simulink model "tqdtqr_rebuild_V3"  (R2021b)
settings: Solver=VariableStepAuto  StartTime=0.0  StopTime=10.0  RelTol=1e-3
undefined symbols (not defined in the file): ATQD_AfterTqMinGain_X_Deg, ATQD_APSCreepBaseTqD_X_kph, ATQD_APSCreepBaseTqD_Y_Deg, ATQD_APSCreepBaseTqR_X_kph, ATQD_APSCreepBaseTqR_Y_Deg, ATQD_APSCreepIterm_X_kph, ATQD_APSCreepIterm_Y_kph, ATQD_APSCreepPterm_X_kph, ATQD_APSCreepPterm_Y_kph, ATQD_APSDecReq_X_kph, ATQD_APSDecReq_Y_mps2, ATQD_APSDecReqCMD_X_kph, ATQD_APSDecReqTs_X_pct, ATQD_APSDecTimeGain_X_Deg, ATQD_APSDecTimeGain_Y_s, ATQD_APSReqLowSpd_X_Deg, ATQD_AutoHoldReleaseBPS_X_Deg, ATQD_AWDLoadTrqnsGain_X_kg, ATQD_AWDLoadTrqnsGain_Y_pct, ATQD_BOSEnBPSPosn_X_kph, ATQD_BOSMap_X_rpm, ATQD_BOSMap_Y_pct, ATQD_CreepBaseTqD_X_kph, ATQD_CreepBaseTqD_Y_Deg, ATQD_CreepBaseTqR_X_kph, ATQD_CreepBaseTqR_Y_Deg, ATQD_CreepBPSDisPosn_X_Deg, ATQD_CreepBPSDisPosnR_X_Deg, ATQD_CreepBPSEnPosn_X_Deg, ATQD_CreepBPSEnPosnR_X_Deg, ATQD_CreepDeltaTq_X_kph, ATQD_CreepIterm_X_kph, ATQD_CreepIterm_Y_kph, ATQD_CreepItermMaxLimit_X_pct, ATQD_CreepPreloadTime_X_kph, ATQD_CreepPreloadTq_X_kph, ATQD_CreepPreloadTq_Y_s, ATQD_CreepProtTq_X_Deg, ATQD_CreepPterm_X_kph, ATQD_CreepPterm_Y_kph, ATQD_CreepRrTqSpRat_X_rpm, ATQD_CreepRrTqSpRat_Y_Nm, ATQD_CreepTargetSpdD_X_pct, ATQD_CreepTargetSpdR_X_pct, ATQD_CreepUpLimitTq_X_rpm, ATQD_DecIneOPDHoldEnDelay_X_Deg, ATQD_DecIneOPDHoldEnDelay_Y_bar, ATQD_ECOTqMapD_X_rpm, ATQD_ECOTqMapD_Y_pct, ATQD_EMTqMapD_X_rpm, ATQD_EMTqMapD_Y_pct, ATQD_EOPDTqMapDCon_X_rpm, ATQD_EOPDTqMapDCon_Y_Deg, ATQD_EstInitVehWeight_X_c, ATQD_FAfterTqCMDGain_X_rpm, ATQD_FAfterTqCMDGain_Y_pct, ATQD_ForceLowSpd_X_Deg, ATQD_ForcePLimitSpd_X_Deg, ATQD_FrLossMAPLowV_X_rpm, ATQD_FrLossMAPLowV_Y_Nm ... (+949)
libraries: simulink x235, hcu_lib x208, tqr x63, tqd x6
(part 3 of 37)

== system tqdtqr_rebuild_V3/SCP_Out ==
  BInpConvert_outputs : Inport
  BMain_outputs : Inport  Port=2
  BOutpConvert_outputs : Inport  Port=3
  Bus Selector : BusSelector  OutputSignals=VTQD_GearActualPosn_enum,VTQD_ParkRequest_flg,VTQD_PBWLockTO_flg,VTQD_PBWUnlockTO_flg,VTQD_TqSourceFr_enum,VTQD_TqSourceRr_enum,VTQD_TqTargetShaftSpd_rpm,VTQD_LimpHomeAct_flg,VTQD_RollRegenEnable_flg,VTQD_EVDriveMode_enum,VTQD_EVDriveModeValid_flg,VTQD_ShiftGearPosn_enum,VTQD_FrActvDmpDisabReq_flg,VTQD_RrActvDmpDisabReq_flg,VTQD_CreepEnable_flg,VTQD_LoSpdBrkCtrl_flg,VTQD_LowIdleAccPedal_flg,VTQD_APSStaSys_enum,VTQD_APSReq_enum,VTQD_APSDecReqA_flg,VTQD_APSDecReq_mps2,VTQD_EstVehWeightResult_kg,VTQD_BOSEnable_flg,VTQD_CreepON_flg,VTQD_PreLoadHold_flg,VTQD_PreLoadPreEn_flg,VTQD_CreepPrLoadEnable_flg,VTQD_RDCActive_enum,VTQD_DriveProtEn_flg,VTQD_ActParkRequest_flg,VTQD_RegenTqLimitEn_flg,VTQD_PedAccTqEn_flg,VTQD_IVIPwrLockSta_enum,VTQD_WhlTqCapGenFr_Nm,VTQD_WhlTqCapGenRr_Nm,VTQD_OPDHoldLamp_flg,VTQD_RegenMode_enum,VTQD_SaveRegenMode_enum,VTQD_FDCVCURegenMode_enum,VTQD_SpdCtrlMode_enum,VTQD_SpdCtrlSta_flg,VTQD_SetSpd_kph,VTQD_SWCCancelSta_flg,VTQD_SWCSetdownSta_flg,VTQD_SWCResUpSta_flg,VTQD_CreepBaseTqD_Nm,VTQD_VehActSpd_kph,VTQD_BrkSwSta_flg,VTQD_SWC2CancelSta_flg,VTQD_SWC2SetdownSta_flg,VTQD_SWC2ResUpSta_flg,VTQD_SWC2LADASSta_flg,VTQD_SpdLim4SetSpd_raw32,VTQD_MaxWhlSlideRate_pct,VTQD_MinWhlSlideRate_pct,VTQD_LeftSlideRate_pct,VTQD_RightSlideRate_pct,VTQD_FrontSlideRate_pct,VTQD_RearSlideRate_pct,VTQD_TrailerDisOPDSta_flg,VTQD_ComboKeyPreEn_flg,VTQD_ComboKeyEn_flg,VTQD_SysMode_enum,VTQD_WhlTqCapMotFr_Nm,VTQD_WhlTqCapMotRr_Nm,VTQD_FrShaftSpd_rpm,VTQD_RrShaftSpd_rpm,VTQD_EPBCarWashMode_flg,VTQD_IVIRockModeEn_flg,VTQD_ForceP_flg,VTQD_SlideRegenLimTq_Nm,VTQD_SimSoundCmd_pct,VTQD_SimSouWaveReq_pct,VTQD_RockModeTCSReq_flg,VTQD_TMEnOutpTqSta_enum,VTQR_RShaftSpdTqLimLow_flg,VTQR_RTimerTqLimLow_flg,VTQR_FShaftSpdTqLimLow_flg,VTQR_FTimerTqLimLow_flg,VTQR_FrFirstOrderInpTs_c,VTQR_RrFirstOrderInpTs_c,VTQR_FrRateLimitInc_Nm,VTQR_FrRateLimitDec_Nm,VTQR_RrRateLimitInc_Nm,VTQR_RrRateLimitDec_Nm,VTQR_FrTqZeroTransLowBound_Nm,VTQR_RrTqZeroTransUpBound_Nm,VTQR_FrTqZeroTrans_enum,VTQR_RrTqZeroTrans_enum
  Bus Selector1 : BusSelector  OutputSignals=VTQD_DriverWhlTqDem_Nm,VTQD_AfterAvailableTqDemFr_Nm,VTQD_AfterAvailableTqDemRr_Nm,VTQD_CoordWhlTqDemFr_Nm,VTQD_CoordWhlTqDemRr_Nm,VTQR_FrTMTqReq_Nm,VTQR_RrTMTqReq_Nm,VTQR_ActualFEDUWhlTqReq_Nm,VTQR_ActualREDUWhlTqReq_Nm,VTQR_NoABSFEDUWhlTqReq_Nm,VTQR_NoABSREDUWhlTqReq_Nm
  Bus Selector2 : BusSelector  OutputSignals=VTQD_FrEDUAvailBrkRgnTq_Nm,VTQD_RrEDUAvailBrkRgnTq_Nm,VTQD_PButtonSta_enum,VTQD_FrRgnDecrSta_flg,VTQD_RrRgnDecrSta_flg,VTQD_DriverWhlTqDemFr_Nm,VTQD_DriverWhlTqDemRr_Nm,VTQD_FrEDUActTq_Nm,VTQD_RrEDUActTq_Nm,VTQD_FrEDURolRgnTq_Nm,VTQD_RrEDURolRgnTq_Nm,VTQD_FrEDUSpd_rpm,VTQD_RrEDUSpd_rpm,VTQD_FrEDUSpdValid_flg,VTQD_FrEDUAvailBrkRgnTqV_flg,VTQD_RrEDUSpdValid_flg,VTQD_RrEDUAvailBrkRgnTqV_flg,VTQD_RgnAbnorSta_flg,VTQD_PTCSPermSta_flg,VTQD_FrRgnPermSta_flg,VTQD_RrRgnPermSta_flg,VTQD_ExternalTqAllow_flg,VTQD_FrIdcMin_A,VTQD_FrIdcMax_A,VTQD_FrUdcMin_V,VTQD_FrUdcMax_V,VTQD_RrIdcMin_A,VTQD_RrIdcMax_A,VTQD_RrUdcMin_V,VTQD_RrUdcMax_V,VTQD_CrashDetd_flg,VTQD_DiagHCrash_flg,VTQD_ReBrakeLPReq_flg,VTQD_ExtShftAllow_flg,VTQD_EquivAccPedalSWSta_flg,VTQD_ExtDoorAllow_flg,VTQD_RegenLimIndSta_flg,VTQD_SetSpdLimWarn_flg,VTQD_CrashUnlockReq_flg,VTQD_CTDCtrl_enum
  Bus Creator : BusCreator  Inputs=140
  BDrivingControl_outputs : Outport
  wires:
  BInpConvert_outputs/1 -> Bus Selector/1
  BMain_outputs/1 -> Bus Selector1/1
  BOutpConvert_outputs/1 -> Bus Selector2/1
  Bus Selector/1 -> Bus Creator/1  "<VTQD_GearActualPosn_enum>"
  Bus Selector/2 -> Bus Creator/2  "<VTQD_ParkRequest_flg>"
  Bus Selector/3 -> Bus Creator/3  "<VTQD_PBWLockTO_flg>"
  Bus Selector/4 -> Bus Creator/4  "<VTQD_PBWUnlockTO_flg>"
  Bus Selector/5 -> Bus Creator/5  "<VTQD_TqSourceFr_enum>"
  Bus Selector/6 -> Bus Creator/6  "<VTQD_TqSourceRr_enum>"
  Bus Selector/7 -> Bus Creator/7  "<VTQD_TqTargetShaftSpd_rpm>"
  Bus Selector/8 -> Bus Creator/8  "<VTQD_LimpHomeAct_flg>"
  Bus Selector/9 -> Bus Creator/9  "<VTQD_RollRegenEnable_flg>"
  Bus Selector/10 -> Bus Creator/10  "<VTQD_EVDriveMode_enum>"
  Bus Selector/11 -> Bus Creator/11  "<VTQD_EVDriveModeValid_flg>"
  Bus Selector/12 -> Bus Creator/12  "<VTQD_ShiftGearPosn_enum>"
  Bus Selector/13 -> Bus Creator/13  "<VTQD_FrActvDmpDisabReq_flg>"
  Bus Selector/14 -> Bus Creator/14  "<VTQD_RrActvDmpDisabReq_flg>"
  Bus Selector/15 -> Bus Creator/15  "<VTQD_CreepEnable_flg>"
  Bus Selector/16 -> Bus Creator/16  "<VTQD_LoSpdBrkCtrl_flg>"
  Bus Selector/17 -> Bus Creator/17  "<VTQD_LowIdleAccPedal_flg>"
  Bus Selector/18 -> Bus Creator/18  "<VTQD_APSStaSys_enum>"
  Bus Selector/19 -> Bus Creator/19  "<VTQD_APSReq_enum>"
  Bus Selector/20 -> Bus Creator/20  "<VTQD_APSDecReqA_flg>"
  Bus Selector/21 -> Bus Creator/21  "<VTQD_APSDecReq_mps2>"
  Bus Selector/22 -> Bus Creator/22  "<VTQD_EstVehWeightResult_kg>"
  Bus Selector/23 -> Bus Creator/23  "<VTQD_BOSEnable_flg>"
  Bus Selector/24 -> Bus Creator/24  "<VTQD_CreepON_flg>"
  Bus Selector/25 -> Bus Creator/25  "<VTQD_PreLoadHold_flg>"
  Bus Selector/26 -> Bus Creator/26  "<VTQD_PreLoadPreEn_flg>"
  Bus Selector/27 -> Bus Creator/27  "<VTQD_CreepPrLoadEnable_flg>"
  Bus Selector/28 -> Bus Creator/28  "<VTQD_RDCActive_enum>"
  Bus Selector/29 -> Bus Creator/29  "<VTQD_DriveProtEn_flg>"
  Bus Selector/30 -> Bus Creator/30  "<VTQD_ActParkRequest_flg>"
  Bus Selector/31 -> Bus Creator/31  "<VTQD_RegenTqLimitEn_flg>"
  Bus Selector/32 -> Bus Creator/32  "<VTQD_PedAccTqEn_flg>"
  Bus Selector/33 -> Bus Creator/33  "<VTQD_IVIPwrLockSta_enum>"
  Bus Selector/34 -> Bus Creator/34  "<VTQD_WhlTqCapGenFr_Nm>"
  Bus Selector/35 -> Bus Creator/35  "<VTQD_WhlTqCapGenRr_Nm>"
  Bus Selector/36 -> Bus Creator/36  "<VTQD_OPDHoldLamp_flg>"
  Bus Selector/37 -> Bus Creator/37  "<VTQD_RegenMode_enum>"
  Bus Selector/38 -> Bus Creator/38  "<VTQD_SaveRegenMode_enum>"
  Bus Selector/39 -> Bus Creator/39  "<VTQD_FDCVCURegenMode_enum>"
  Bus Selector/40 -> Bus Creator/40  "<VTQD_SpdCtrlMode_enum>"
  Bus Selector/41 -> Bus Creator/41  "<VTQD_SpdCtrlSta_flg>"
  Bus Selector/42 -> Bus Creator/42  "<VTQD_SetSpd_kph>"
  Bus Selector/43 -> Bus Creator/43  "<VTQD_SWCCancelSta_flg>"
  Bus Selector/44 -> Bus Creator/44  "<VTQD_SWCSetdownSta_flg>"
  Bus Selector/45 -> Bus Creator/45  "<VTQD_SWCResUpSta_flg>"
  Bus Selector/46 -> Bus Creator/46  "<VTQD_CreepBaseTqD_Nm>"
  Bus Selector/47 -> Bus Creator/47  "<VTQD_VehActSpd_kph>"
  Bus Selector/48 -> Bus Creator/48  "<VTQD_BrkSwSta_flg>"
  Bus Selector/49 -> Bus Creator/49  "<VTQD_SWC2CancelSta_flg>"
  Bus Selector/50 -> Bus Creator/50  "<VTQD_SWC2SetdownSta_flg>"
  Bus Selector/51 -> Bus Creator/51  "<VTQD_SWC2ResUpSta_flg>"
  Bus Selector/52 -> Bus Creator/52  "<VTQD_SWC2LADASSta_flg>"
  Bus Selector/53 -> Bus Creator/53  "<VTQD_SpdLim4SetSpd_raw32>"
  Bus Selector/54 -> Bus Creator/54  "<VTQD_MaxWhlSlideRate_pct>"
  Bus Selector/55 -> Bus Creator/55  "<VTQD_MinWhlSlideRate_pct>"
  Bus Selector/56 -> Bus Creator/56  "<VTQD_LeftSlideRate_pct>"
  Bus Selector/57 -> Bus Creator/57  "<VTQD_RightSlideRate_pct>"
  Bus Selector/58 -> Bus Creator/58  "<VTQD_FrontSlideRate_pct>"
  Bus Selector/59 -> Bus Creator/59  "<VTQD_RearSlideRate_pct>"
  Bus Selector/60 -> Bus Creator/60  "<VTQD_TrailerDisOPDSta_flg>"
  Bus Selector/61 -> Bus Creator/61  "<VTQD_ComboKeyPreEn_flg>"
  Bus Selector/62 -> Bus Creator/62  "<VTQD_ComboKeyEn_flg>"
  Bus Selector/63 -> Bus Creator/63  "<VTQD_SysMode_enum>"
  Bus Selector/64 -> Bus Creator/64  "<VTQD_WhlTqCapMotFr_Nm>"
  Bus Selector/65 -> Bus Creator/65  "<VTQD_WhlTqCapMotRr_Nm>"
  Bus Selector/66 -> Bus Creator/66  "<VTQD_FrShaftSpd_rpm>"
  Bus Selector/67 -> Bus Creator/67  "<VTQD_RrShaftSpd_rpm>"
  Bus Selector/68 -> Bus Creator/68  "<VTQD_EPBCarWashMode_flg>"
  Bus Selector/69 -> Bus Creator/69  "<VTQD_IVIRockModeEn_flg>"
  Bus Selector/70 -> Bus Creator/70  "<VTQD_ForceP_flg>"
  Bus Selector/71 -> Bus Creator/71  "<VTQD_SlideRegenLimTq_Nm>"
  Bus Selector/72 -> Bus Creator/72  "<VTQD_SimSoundCmd_pct>"
  Bus Selector/73 -> Bus Creator/73  "<VTQD_SimSouWaveReq_pct>"
  Bus Selector/74 -> Bus Creator/74  "<VTQD_RockModeTCSReq_flg>"
  Bus Selector/75 -> Bus Creator/75  "<VTQD_TMEnOutpTqSta_enum>"
  Bus Selector1/1 -> Bus Creator/90  "<VTQD_DriverWhlTqDem_Nm>"
  Bus Selector1/2 -> Bus Creator/91  "<VTQD_AfterAvailableTqDemFr_Nm>"
  Bus Selector1/3 -> Bus Creator/92  "<VTQD_AfterAvailableTqDemRr_Nm>"
  Bus Selector1/4 -> Bus Creator/93  "<VTQD_CoordWhlTqDemFr_Nm>"
  Bus Selector1/5 -> Bus Creator/94  "<VTQD_CoordWhlTqDemRr_Nm>"
  Bus Selector2/1 -> Bus Creator/101  "<VTQD_FrEDUAvailBrkRgnTq_Nm>"
  Bus Selector2/2 -> Bus Creator/102  "<VTQD_RrEDUAvailBrkRgnTq_Nm>"
  Bus Selector2/3 -> Bus Creator/103  "<VTQD_PButtonSta_enum>"
  Bus Selector2/4 -> Bus Creator/104  "<VTQD_FrRgnDecrSta_flg>"
  Bus Selector2/5 -> Bus Creator/105  "<VTQD_RrRgnDecrSta_flg>"
  Bus Selector2/6 -> Bus Creator/106  "<VTQD_DriverWhlTqDemFr_Nm>"
  Bus Selector2/7 -> Bus Creator/107  "<VTQD_DriverWhlTqDemRr_Nm>"
  Bus Selector2/8 -> Bus Creator/108  "<VTQD_FrEDUActTq_Nm>"
  Bus Selector2/9 -> Bus Creator/109  "<VTQD_RrEDUActTq_Nm>"
  Bus Selector2/10 -> Bus Creator/110  "<VTQD_FrEDURolRgnTq_Nm>"
  Bus Selector2/11 -> Bus Creator/111  "<VTQD_RrEDURolRgnTq_Nm>"
  Bus Selector2/12 -> Bus Creator/112  "<VTQD_FrEDUSpd_rpm>"
  Bus Selector2/13 -> Bus Creator/113  "<VTQD_RrEDUSpd_rpm>"
  Bus Selector2/14 -> Bus Creator/114  "<VTQD_FrEDUSpdValid_flg>"
  Bus Selector2/15 -> Bus Creator/115  "<VTQD_FrEDUAvailBrkRgnTqV_flg>"
  Bus Selector2/16 -> Bus Creator/116  "<VTQD_RrEDUSpdValid_flg>"
  Bus Selector2/17 -> Bus Creator/117  "<VTQD_RrEDUAvailBrkRgnTqV_flg>"
  Bus Selector2/18 -> Bus Creator/118  "<VTQD_RgnAbnorSta_flg>"
  Bus Selector2/19 -> Bus Creator/119  "<VTQD_PTCSPermSta_flg>"
  Bus Selector2/20 -> Bus Creator/120  "<VTQD_FrRgnPermSta_flg>"
  Bus Selector2/21 -> Bus Creator/121  "<VTQD_RrRgnPermSta_flg>"
  Bus Selector2/22 -> Bus Creator/122  "<VTQD_ExternalTqAllow_flg>"
  Bus Selector2/23 -> Bus Creator/123  "<VTQD_FrIdcMin_A>"
  Bus Selector2/24 -> Bus Creator/124  "<VTQD_FrIdcMax_A>"
  Bus Selector2/25 -> Bus Creator/125  "<VTQD_FrUdcMin_V>"
  Bus Selector2/26 -> Bus Creator/126  "<VTQD_FrUdcMax_V>"
  Bus Selector2/27 -> Bus Creator/127  "<VTQD_RrIdcMin_A>"
  Bus Selector2/28 -> Bus Creator/128  "<VTQD_RrIdcMax_A>"
  Bus Selector2/29 -> Bus Creator/129  "<VTQD_RrUdcMin_V>"
  Bus Selector2/30 -> Bus Creator/130  "<VTQD_RrUdcMax_V>"
  Bus Selector2/31 -> Bus Creator/131  "<VTQD_CrashDetd_flg>"
  Bus Selector2/32 -> Bus Creator/132  "<VTQD_DiagHCrash_flg>"
  Bus Selector2/33 -> Bus Creator/133  "<VTQD_ReBrakeLPReq_flg>"
  Bus Selector2/34 -> Bus Creator/134  "<VTQD_ExtShftAllow_flg>"
  Bus Selector2/35 -> Bus Creator/135  "<VTQD_EquivAccPedalSWSta_flg>"
  Bus Selector2/36 -> Bus Creator/136  "<VTQD_ExtDoorAllow_flg>"
  Bus Selector2/37 -> Bus Creator/137  "<VTQD_RegenLimIndSta_flg>"
  Bus Selector2/38 -> Bus Creator/138  "<VTQD_SetSpdLimWarn_flg>"
  Bus Creator/1 -> BDrivingControl_outputs/1
  Bus Selector/76 -> Bus Creator/76  "<VTQR_RShaftSpdTqLimLow_flg>"
  Bus Selector/77 -> Bus Creator/77  "<VTQR_RTimerTqLimLow_flg>"
  Bus Selector/78 -> Bus Creator/78  "<VTQR_FShaftSpdTqLimLow_flg>"
  Bus Selector/79 -> Bus Creator/79  "<VTQR_FTimerTqLimLow_flg>"
  Bus Selector/80 -> Bus Creator/80  "<VTQR_FrFirstOrderInpTs_c>"
  Bus Selector/81 -> Bus Creator/81  "<VTQR_RrFirstOrderInpTs_c>"
  Bus Selector/82 -> Bus Creator/82  "<VTQR_FrRateLimitInc_Nm>"
  Bus Selector/83 -> Bus Creator/83  "<VTQR_FrRateLimitDec_Nm>"
  Bus Selector/84 -> Bus Creator/84  "<VTQR_RrRateLimitInc_Nm>"
  Bus Selector/85 -> Bus Creator/85  "<VTQR_RrRateLimitDec_Nm>"
  Bus Selector/86 -> Bus Creator/86  "<VTQR_FrTqZeroTransLowBound_Nm>"
  Bus Selector/87 -> Bus Creator/87  "<VTQR_RrTqZeroTransUpBound_Nm>"
  Bus Selector/88 -> Bus Creator/88  "<VTQR_FrTqZeroTrans_enum>"
  Bus Selector/89 -> Bus Creator/89  "<VTQR_RrTqZeroTrans_enum>"
  Bus Selector1/6 -> Bus Creator/95  "<VTQR_FrTMTqReq_Nm>"
  Bus Selector1/7 -> Bus Creator/96  "<VTQR_RrTMTqReq_Nm>"
  Bus Selector1/8 -> Bus Creator/97  "<VTQR_ActualFEDUWhlTqReq_Nm>"
  Bus Selector1/9 -> Bus Creator/98  "<VTQR_ActualREDUWhlTqReq_Nm>"
  Bus Selector1/10 -> Bus Creator/99  "<VTQR_NoABSFEDUWhlTqReq_Nm>"
  Bus Selector1/11 -> Bus Creator/100  "<VTQR_NoABSREDUWhlTqReq_Nm>"
  Bus Selector2/39 -> Bus Creator/139  "<VTQD_CrashUnlockReq_flg>"
  Bus Selector2/40 -> Bus Creator/140  "<VTQD_CTDCtrl_enum>"

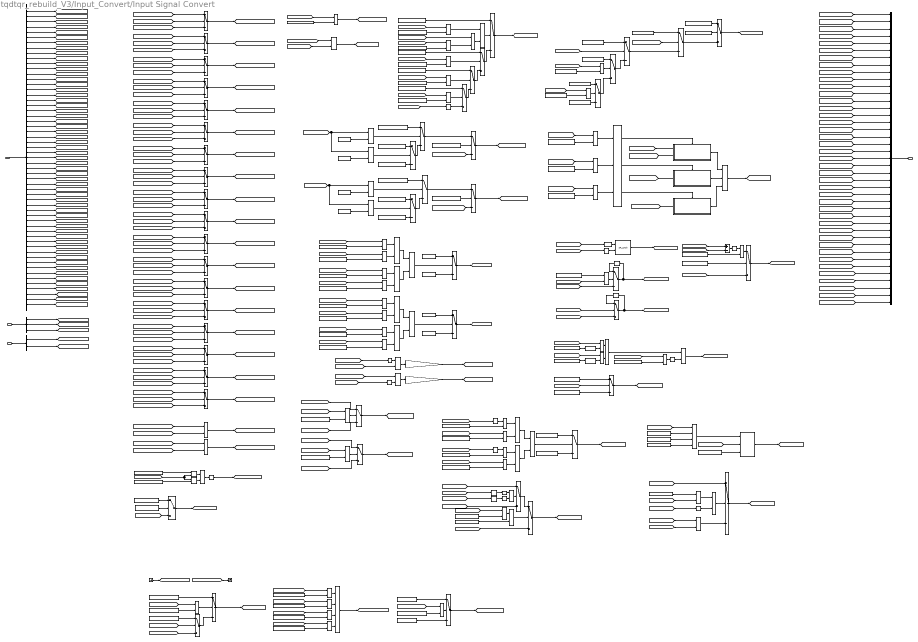
== system tqdtqr_rebuild_V3/Input_Convert/Input Signal Convert ==
  note: Creep function switch2
  note: Calculate vehicle actual speed
  note: CAN4 SWC SCP
  note: CAN3 MCU SCP
  note: Rolling Regen Cancel Request Handle
  note: Brake pedal signal handle
  note: Actual gear position signal defination converter for CAN bus
  note: Fr and Rr Wheel Rotate Diraction Detect
  note: Fr and Rr Wheel Rotate Diraction Detect
  note: Target Shaft Speed and Direction Judgement
  note: %VINP_IVIPWModeReq_enum
      | ENUM_IVIPWMODEREQ_NRM = uint8( 0 );
      | ENUM_IVIPWMODEREQ_SPORT = uint8( 1 );
      | ENUM_IVIPWMODEREQ_ECO = uint8( 2 ); ENUM_IVIPWMODEREQ_NOREQUEST = uint8( 3 );
  note: % VTQD_EVDriveMode_enum
      | ENUM_DRIVEMODE_NRM = uint8( 0 );
      | ENUM_DRIVEMODE_ECO = uint8( 1 );
      | ENUM_DRIVEMODE_SPORT = uint8( 2 );
      | ENUM_DRIVEMODE_SNOW = uint8( 3 );
  note: Driving mode determination
  note: MCU Ready for External judgement
  note: Regen Mode Latch
  note: Exhibition Status
  note: Check gear position(for tq coordination)
  BSCPIn_outputs : Inport
  BFunction_outputs : Inport  Port=2
  BMain_outputs : Inport  Port=3
  AND : Logic  Inputs=4  AllPortsSameDT=off  OutDataTypeStr=boolean
  AND{1,3..4,9,18} (5 alike) : Logic  AllPortsSameDT=off  OutDataTypeStr=boolean
  AND10 : Logic  Operator=OR  AllPortsSameDT=off  OutDataTypeStr=boolean
  AWDMCUReadyExt_flg : Subsystem  TreatAsAtomicUnit=on
  Abs{,1..4} (5 alike) : Abs
  Add : Sum  Inputs=+-
  Bus Selector : BusSelector  OutputSignals=task_time_s,VTQD_ActAPSPosn_pct,VTQD_LowIdleAccPedal_flg,VPMM_DrivetrainSelect_enum,VINP_IVIPWModeReq_enum,VINP_IVISnowModeCmd_flg,VINP_CANMsgValidMCUNR1_flg,VINP_FrEDURotateDirctionNidec_enum,VINP_FrEDURotateDirction_enum,VINP_RrEDURotateDirctionNidec_enum,VINP_RrEDURotateDirction_enum,VINP_FrTMSpdNidec_rpm,VINP_FrTMSpd_rpm,VINP_RrTMSpdNidec_rpm,VINP_RrTMSpd_rpm,VINP_FrRegenAvailTqNidec_Nm,VINP_FrRegenAvailTq_Nm,VINP_RrRegenAvailTqNidec_Nm,VINP_RrRegenAvailTq_Nm,VINP_FrEDURealTMTqNidec_Nm,VINP_FrEDURealTMTq_Nm,VINP_RrEDURealTMTqNidec_Nm,VINP_RrEDURealTMTq_Nm,VINP_FrMotorAvailTqNidec_Nm,VINP_FrMotorAvailTq_Nm,VINP_RrMotorAvailTqNidec_Nm,VINP_RrMotorAvailTq_Nm,VINP_MCUWarnFNidec_enum,VINP_MCUWarnF_enum,VINP_MCUWarnRNidec_enum,VINP_MCUWarnR_enum,VINP_FrMCUDCBusVoltNidec_V,VINP_FrMCUDCBusVolt_V,VINP_RrMCUDCBusVoltNidec_V,VINP_RrMCUDCBusVolt_V,VINP_FrMCUTempNidec_C,VINP_FrMCUTemp_C,VINP_FrTMTempNidec_C,VINP_FrTMTemp_C,VINP_RrMCUTempNidec_C,VINP_RrMCUTemp_C,VINP_RrTMTempNidec_C,VINP_RrTMTemp_C,VINP_SWCRegenUp_flg,VINP_SWC2LRegenUpSta_flg,VINP_SWC2RRegenDownSta_flg,VINP_SWCRegenDown_flg,VTQD_RDCActive_enum,VINP_BrakeSWGPIO_flg,VTQD_LimpHomeAct_flg,VINP_BrkSwSta_flg,VVMC_APSActive_flg,VINP_VehSpeed_kph,VTQD_ActAPSPosn_pct,VINP_DIDGetExhibitMode_enum,VINP_EPBSta_enum,VINP_IVICreepSWReq_flg
  Bus Selector1 : BusSelector  OutputSignals=VTQD_GearActualPosn_enum,VTQD_FDCVCURegenMode_enum,VTQD_OPDHoldForceEn_flg
  Bus Selector2 : BusSelector  OutputSignals=VTQR_NoABSFEDUWhlTqReq_Nm,VTQR_NoABSREDUWhlTqReq_Nm
  Bus Creator : BusCreator  Inputs=41
  Constant : Constant  Value=KTQD_CreepSW_flg_ovrdflg
  Constant1 : Constant  Value=KTQD_RgnModeChgResetSW_flg
  Constant{9..10,29,43,53} (5 alike) : Constant  Value=ENUM_GEARACTUALPOSN_D
  Constant{11,13..14,30,35} (5 alike) : Constant  Value=ENUM_TMROTATEDIRECTACT_REVERSE  OutDataTypeStr=Inherit: Inherit via back propagation
  Constant116 : Constant  Value=0xBB
  Constant12 : Constant  Value=ENUM_TMROTATEDIRECTACT_STOP  OutDataTypeStr=Inherit: Inherit via back propagation
  Constant130 : Constant  Value=ENUM_DRIVEMODE_SNOW
  Constant132 : Constant  Value=ENUM_DRIVEMODE_NRM
  Constant15 : Constant  Value=ENUM_TMROTATEDIRECTACT_STOP  OutDataTypeStr=Inherit: Inherit via back propagation
  Constant16 : Constant  Value=KTQD_DriveModeReq_enum_ovrdflg  OutDataTypeStr=Inherit: Inherit via back propagation
  Constant17 : Constant  Value=KTQD_DriveModeReq_enum_ovrdval  OutDataTypeStr=Inherit: Inherit via back propagation
  Constant{5,18,20,23} (4 alike) : Constant  Value=ZERO_FLOAT  OutDataTypeStr=Inherit: Inherit via back propagation
  Constant19 : Constant  Value=KTQD_AbsoluteMotorSpdDir_flg  OutDataTypeStr=Inherit: Inherit via back propagation
  Constant2 : Constant  Value=ENUM_RDCACTSTA_NOREQUEST
  Constant21 : Constant  Value=ENUM_DRIVETRAIN_FWD
  Constant22 : Constant  Value=KTQD_AbsoluteMotorSpdDir_flg  OutDataTypeStr=Inherit: Inherit via back propagation
  Constant{24,31,36,42,56} (5 alike) : Constant  Value=ENUM_GEARACTUALPOSN_R
  Constant{7,25,28,32,37} (5 alike) : Constant  Value=ENUM_TMROTATEDIRECTACT_FORWARD  OutDataTypeStr=Inherit: Inherit via back propagation
  Constant26 : Constant  Value=KTQD_VehActSpdNegGain_gain
  Constant27 : Constant  Value=KTQD_VehActSpdPosGain_gain
  Constant3 : Constant  Value=RPM2RADPS
  Constant33 : Constant  Value=ONE_FLOAT
  Constant34 : Constant  Value=MINUSONE_FLOAT
  Constant38 : Constant  Value=ONE_FLOAT
  Constant39 : Constant  Value=MINUSONE_FLOAT
  Constant4 : Constant  Value=KTQD_TireRadius_m
  Constant40 : Constant  Value=KTQD_RPM2VehSpdTs_c
  Constant41 : Constant  Value=KTQD_ActSpdInpSourSW_flg
  Constant44 : Constant  Value=ENUM_REGENLEVEL_LV1
  Constant45 : Constant  Value=MINUSONE_FLOAT
  Constant46 : Constant  Value=ENUM_DRIVEMODE_NRM
  Constant47 : Constant  Value=ENUM_IVIPWMODEREQ_SPORT
  Constant48 : Constant  Value=KTQD_CreepVehSpdSW_flg
  Constant49 : Constant  Value=ENUM_DRIVEMODE_SPORT
  Constant50 : Constant  Value=ENUM_GEARPOSNTOCAN_N  OutDataTypeStr=Inherit: Inherit via back propagation
  Constant51 : Constant  Value=ENUM_GEARPOSNTOCAN_D  OutDataTypeStr=Inherit: Inherit via back propagation
  Constant52 : Constant  Value=ENUM_EPBSTA_APPLIED
  Constant54 : Constant  Value=ENUM_GEARACTUALPOSN_N
  Constant55 : Constant  Value=ENUM_GEARPOSNTOCAN_R  OutDataTypeStr=Inherit: Inherit via back propagation
  Constant57 : Constant  Value=ENUM_GEARPOSNTOCAN_P  OutDataTypeStr=Inherit: Inherit via back propagation
  Constant58 : Constant  Value=ENUM_GEARACTUALPOSN_P
  Constant59 : Constant  Value=KTQR_LaunchEnPedal_pct
  Constant6 : Constant  Value=ENUM_DRIVETRAIN_FWD
  Constant60 : Constant  Value=KTQR_LaunchEnSpd_kph
  Constant61 : Constant  Value=ONE_FLOAT
  Constant62 : Constant  Value=KTQD_CreepSW_flg_ovrdval
  Constant66 : Constant  Value=ENUM_DRIVETRAIN_AWD
  Constant69 : Constant  Value=ENUM_DRIVEMODE_ECO
  Constant70 : Constant  Value=ENUM_IVIPWMODEREQ_ECO
  Constant71 : Constant  Value=ENUM_DRIVEMODE_SPORT
  Constant72 : Constant  Value=ENUM_DRIVETRAIN_RWD
  Constant73 : Constant  Value=KTQD_RgnModeChgResetAPSDev_pct
  Constant74 : Constant  Value=KTQD_RgnModeChgSW_flg
  Constant75 : Constant  Value=ENUM_DRIVETRAIN_AWD
  Constant76 : Constant  Value=ENUM_DRIVETRAIN_FWD
  Constant8 : Constant  Value=MPS2KPH
  Constant81 : Constant  Value=ENUM_GEARACTUALPOSN_P
  Constant96 : Constant  Value=0xAA
  Constant97 : Constant  Value=ENUM_PWRLOCKSta_LOCKED
  Constant98 : Constant  Value=ENUM_PWRLOCKSta_UNLOCKED
  Data Type Conversion3 : DataTypeConversion  OutDataTypeStr=uint8
  Data Type Conversion8 : DataTypeConversion  OutDataTypeStr=uint8
  Delay : Delay  DelayLength=1  InitialCondition=single(0)
      settings: AttributesFormatString=%<InitialCondition>
  Delay1 : Delay  DelayLength=1  InitialCondition=uint8(0)
      settings: AttributesFormatString=%<InitialCondition>
  Delay2 : Delay  DelayLength=1  InitialCondition=single(0.0)
      settings: AttributesFormatString=%<InitialCondition>
  Delay3 : Delay  DelayLength=1
  Delay4 : Delay  DelayLength=1  InitialCondition=boolean(0)
      settings: AttributesFormatString=%<InitialCondition>
  Delay5 : Delay  DelayLength=1  InitialCondition=uint8(0)
      settings: AttributesFormatString=%<InitialCondition>
  Delay6 : Delay  DelayLength=1  InitialCondition=uint8(0)
      settings: AttributesFormatString=%<InitialCondition>
  Delay7 : Delay  DelayLength=1  InitialCondition=ENUM_GEARPOSNTOCAN_FAIL
      settings: AttributesFormatString=%<InitialCondition>
  Delay8 : Delay  DelayLength=1  InitialCondition=single(0)
      settings: AttributesFormatString=%<InitialCondition>
  Detect Change : simulink/Logic and Bit Operations/Detect Change  vinit=boolean(0)  OutDataTypeStr=boolean
  Equal{,1..19,21..29,31,34,47..48,51} (34 alike) : RelationalOperator  Operator===  OutDataTypeStr=boolean  RndMeth=Simplest
  Equal20 : RelationalOperator  Operator=~=  OutDataTypeStr=boolean  RndMeth=Simplest
  FWDMCUReadyExt_flg : Subsystem  TreatAsAtomicUnit=on
  FirstOrderFilter : hcu_lib/Basic_Blocks/FirstOrderFilter
  Gain : Gain  Gain=1/KTQD_FrTMTotalGearRatio_gain
  Gain2 : Gain  Gain=1/KTQD_RrTMTotalGearRatio_gain
  GreaterThan : RelationalOperator  Operator=>  OutDataTypeStr=boolean  RndMeth=Simplest
  GreaterThan1 : RelationalOperator  Operator=<  OutDataTypeStr=boolean  RndMeth=Simplest
  GreaterThan2 : RelationalOperator  Operator=>  OutDataTypeStr=boolean  RndMeth=Simplest
  GreaterThan3 : RelationalOperator  Operator=<  OutDataTypeStr=boolean  RndMeth=Simplest
  Ground1 : Ground
  If : If  NumInputs=3  IfExpression=u1 ~= 0  ElseIfExpressions=u2 ~= 0
  LiuzgSwitch{1..5,7..13,21..22,24} (15 alike) : Switch  Criteria=u2 ~= 0
      settings: AttributesFormatString=<%<Criteria>>
  Logical Operator{,2..3,5..6,8} (6 alike) : Logic  AllPortsSameDT=off  OutDataTypeStr=boolean
  Logical Operator1 : Logic  Operator=OR  AllPortsSameDT=off  OutDataTypeStr=boolean
  Logical Operator4 : Logic  Operator=OR  AllPortsSameDT=off  OutDataTypeStr=boolean
  Logical Operator7 : Logic  Operator=OR  AllPortsSameDT=off  OutDataTypeStr=boolean
  Merge : Merge  Inputs=3
  NOT1 : Logic  Operator=NOT  AllPortsSameDT=off  OutDataTypeStr=boolean
  OR{,1..4,6} (6 alike) : Logic  Operator=OR  AllPortsSameDT=off  OutDataTypeStr=boolean
  Product : Product
  Product1 : Product  Inputs=4
  Product2 : Product
  Product3 : Product
  RWDMCUReadyExt_flg : Subsystem  TreatAsAtomicUnit=on
  RegenLV_inc1 : Constant  Value=ENUM_GEARACTUALPOSN_R
  RegenLV_inc2 : Constant  Value=ENUM_DRIVEMODE_ECO
  RegenLV_inc5 : Constant  Value=ENUM_GEARACTUALPOSN_R
  RegenLV_inc6 : Constant  Value=ENUM_DRIVEMODE_NRM
  Relational Operator1 : RelationalOperator  Operator=>  OutDataTypeStr=boolean  RndMeth=Simplest
  Relational Operator2 : RelationalOperator  Operator=>  OutDataTypeStr=boolean  RndMeth=Simplest
  Relational Operator4 : RelationalOperator  Operator=>  OutDataTypeStr=boolean  RndMeth=Simplest
  Relational Operator6 : RelationalOperator  Operator=<=  OutDataTypeStr=boolean  RndMeth=Simplest
  Relay1 : Relay  OnSwitchValue=KTQD_CreepDisVehSpd_kph  OffSwitchValue=KTQD_CreepEnVehSpd_kph  OnOutputValue=0  OffOutputValue=1  OutDataTypeStr=boolean
      settings: AttributesFormatString=|
      | Off: %<OffSwitchValue>
      | On: %<OnSwitchValue>
  SR_Latch : hcu_lib/Basic_Blocks/SR_Latch
  Switch{,1..17,23..33} (29 alike) : Switch  Criteria=u2 ~= 0
      Switch settings: AttributesFormatString=%<Criteria>
      Switch1 settings: AttributesFormatString=%<Criteria>
      Switch10 settings: AttributesFormatString=%<Criteria>
      Switch11 settings: AttributesFormatString=%<Criteria>
      Switch12 settings: AttributesFormatString=%<Criteria>
      Switch13 settings: AttributesFormatString=%<Criteria>
      Switch14 settings: AttributesFormatString=%<Criteria>
      Switch15 settings: AttributesFormatString=%<Criteria>
      Switch16 settings: AttributesFormatString=%<Criteria>
      Switch17 settings: AttributesFormatString=%<Criteria>
      Switch2 settings: AttributesFormatString=%<Criteria>
      Switch23 settings: AttributesFormatString=%<Criteria>
      Switch24 settings: AttributesFormatString=%<Criteria>
      Switch25 settings: AttributesFormatString=%<Criteria>
      Switch26 settings: AttributesFormatString=%<Criteria>
      Switch28 settings: AttributesFormatString=%<Criteria>
      Switch29 settings: AttributesFormatString=%<Criteria>
      Switch3 settings: AttributesFormatString=%<Criteria>
      Switch30 settings: AttributesFormatString=%<Criteria>
      Switch31 settings: AttributesFormatString=%<Criteria>
      Switch32 settings: AttributesFormatString=%<Criteria>
      Switch33 settings: AttributesFormatString=%<Criteria>
      Switch4 settings: AttributesFormatString=%<Criteria>
      Switch5 settings: AttributesFormatString=%<Criteria>
      Switch6 settings: AttributesFormatString=%<Criteria>
      Switch7 settings: AttributesFormatString=%<Criteria>
      Switch8 settings: AttributesFormatString=%<Criteria>
      Switch9 settings: AttributesFormatString=%<Criteria>
  Switch{18..22} (5 alike) : Switch  Criteria=u2 ~= 0  Threshold=0.5
      settings: AttributesFormatString=%<Criteria>
  Terminator2 : Terminator
  BSignalConvert_outputs : Outport
  wires:
  Switch10/1 -> [VTQD_SCPMCUWarnF_enum]  "VTQD_SCPMCUWarnF_enum"
  Bus Selector/8 -> [VINP_FrEDURotateDirctionNidec_enum]  "<VINP_FrEDURotateDirctionNidec_enum>"
  Bus Selector/7 -> [VINP_CANMsgValidMCUNR1_flg]  "<VINP_CANMsgValidMCUNR1_flg>"
  Bus Selector/23 -> [VINP_RrEDURealTMTq_Nm]  "<VINP_RrEDURealTMTq_Nm>"
  Switch/1 -> [VTQD_SCPFrEDURotateDirction_enum]  "VTQD_SCPFrEDURotateDirction_enum"
  Bus Selector/9 -> [VINP_FrEDURotateDirction_enum]  "<VINP_FrEDURotateDirction_enum>"
  Bus Selector/42 -> [VINP_RrTMTempNidec_C]  "<VINP_RrTMTempNidec_C>"
  Bus Selector/18 -> [VINP_RrRegenAvailTqNidec_Nm]  "<VINP_RrRegenAvailTqNidec_Nm>"
  Bus Selector/22 -> [VINP_RrEDURealTMTqNidec_Nm]  "<VINP_RrEDURealTMTqNidec_Nm>"
  Bus Selector/14 -> [VINP_RrTMSpdNidec_rpm]  "<VINP_RrTMSpdNidec_rpm>"
  Switch6/1 -> [VTQD_SCPFrEDURealTMTq_Nm]  "VTQD_SCPFrEDURealTMTq_Nm"
  Bus Selector/34 -> [VINP_RrMCUDCBusVoltNidec_V]  "<VINP_RrMCUDCBusVoltNidec_V>"
  Bus Selector/50 -> [VTQD_LimpHomeAct_flg]  "<VTQD_LimpHomeAct_flg>"
  Bus Selector/31 -> [VINP_MCUWarnR_enum]  "<VINP_MCUWarnR_enum>"
  Bus Selector/16 -> [VINP_FrRegenAvailTqNidec_Nm]  "<VINP_FrRegenAvailTqNidec_Nm>"
  Bus Selector/21 -> [VINP_FrEDURealTMTq_Nm]  "<VINP_FrEDURealTMTq_Nm>"
  [VINP_SWC2LRegenUpSta_flg] -> OR/2
  [VINP_RrEDURotateDirction_enum] -> Switch1/3
  [VINP_FrEDURotateDirctionNidec_enum] -> Switch/1
  [VINP_FrMCUTempNidec_C] -> Switch14/1
  Bus Selector/49 -> [VINP_BrakeSWGPIO_flg]  "<VINP_BrakeSWGPIO_flg>"
  Bus Selector/10 -> [VINP_RrEDURotateDirctionNidec_enum]  "<VINP_RrEDURotateDirctionNidec_enum>"
  [VINP_MCUWarnFNidec_enum] -> Switch10/1
  Bus Selector/33 -> [VINP_FrMCUDCBusVolt_V]  "<VINP_FrMCUDCBusVolt_V>"
  Switch12/1 -> [VTQD_SCPFrMCUDCBusVolt_V]  "VTQD_SCPFrMCUDCBusVolt_V"
  [VINP_RrMCUDCBusVolt_V] -> Switch13/3
  [VINP_CANMsgValidMCUNR1_flg] -> Switch8/2
  [VINP_RrEDURotateDirctionNidec_enum] -> Switch1/1
  Bus Selector/48 -> [VTQD_RDCActive_enum]  "<VTQD_RDCActive_enum>"
  Bus Selector/47 -> [VINP_SWCRegenDown_flg]  "<VINP_SWCRegenDown_flg>"
  Bus Selector/44 -> [VINP_SWCRegenUp_flg]  "<VINP_SWCRegenUp_flg>"
  [VINP_RrEDURealTMTq_Nm] -> Switch7/3
  [VINP_RrTMTemp_C] -> Switch17/3
  [VINP_CANMsgValidMCUNR1_flg] -> Switch17/2
  [VINP_FrEDURotateDirction_enum] -> Switch/3
  Bus Selector/45 -> [VINP_SWC2LRegenUpSta_flg]  "<VINP_SWC2LRegenUpSta_flg>"
  [VINP_FrMCUDCBusVoltNidec_V] -> Switch12/1
  Bus Selector/38 -> [VINP_FrTMTempNidec_C]  "<VINP_FrTMTempNidec_C>"
  Bus Selector/35 -> [VINP_RrMCUDCBusVolt_V]  "<VINP_RrMCUDCBusVolt_V>"
  Bus Selector/28 -> [VINP_MCUWarnFNidec_enum]  "<VINP_MCUWarnFNidec_enum>"
  Bus Selector/27 -> [VINP_RrMotorAvailTq_Nm]  "<VINP_RrMotorAvailTq_Nm>"
  OR1/1 -> [VTQD_SCPSWCRegenDown_flg]  "VTQD_SCPSWCRegenDown_flg"
  Bus Selector/36 -> [VINP_FrMCUTempNidec_C]  "<VINP_FrMCUTempNidec_C>"
  Bus Selector/37 -> [VINP_FrMCUTemp_C]  "<VINP_FrMCUTemp_C>"
  [VINP_RrEDURealTMTqNidec_Nm] -> Switch7/1
  Bus Selector/30 -> [VINP_MCUWarnRNidec_enum]  "<VINP_MCUWarnRNidec_enum>"
  Bus Selector/40 -> [VINP_RrMCUTempNidec_C]  "<VINP_RrMCUTempNidec_C>"
  Bus Selector/32 -> [VINP_FrMCUDCBusVoltNidec_V]  "<VINP_FrMCUDCBusVoltNidec_V>"
  Bus Selector/25 -> [VINP_FrMotorAvailTq_Nm]  "<VINP_FrMotorAvailTq_Nm>"
  Bus Selector/39 -> [VINP_FrTMTemp_C]  "<VINP_FrTMTemp_C>"
  Switch17/1 -> [VTQD_SCPRrTMTemp_C]  "VTQD_SCPRrTMTemp_C"
  [VINP_FrTMTempNidec_C] -> Switch15/1
  [VINP_MCUWarnR_enum] -> Switch11/3
  [VINP_FrMCUTemp_C] -> Switch14/3
  [VINP_FrTMTemp_C] -> Switch15/3
  [VINP_RrMCUTemp_C] -> Switch16/3
  [VINP_CANMsgValidMCUNR1_flg] -> Switch16/2
  [VINP_CANMsgValidMCUNR1_flg] -> Switch12/2
  [VINP_RrMCUTempNidec_C] -> Switch16/1
  [VINP_FrMCUDCBusVolt_V] -> Switch12/3
  Switch13/1 -> [VTQD_SCPRrMCUDCBusVolt_V]  "VTQD_SCPRrMCUDCBusVolt_V"
  [VINP_CANMsgValidMCUNR1_flg] -> Switch13/2
  OR/1 -> [VTQD_SCPSWCRegenUp_flg]  "VTQD_SCPSWCRegenUp_flg"
  [VINP_CANMsgValidMCUNR1_flg] -> Switch9/2
  [VINP_FrMotorAvailTqNidec_Nm] -> Switch8/1
  [VINP_CANMsgValidMCUNR1_flg] -> Switch7/2
  [VINP_FrRegenAvailTqNidec_Nm] -> Switch4/1
  Switch9/1 -> [VTQD_SCPRrMotorAvailTq_Nm]  "VTQD_SCPRrMotorAvailTq_Nm"
  [VINP_RrMotorAvailTqNidec_Nm] -> Switch9/1
  Switch8/1 -> [VTQD_SCPFrMotorAvailTq_Nm]  "VTQD_SCPFrMotorAvailTq_Nm"
  Switch5/1 -> [VTQD_SCPRrRegenAvailTq_Nm]  "VTQD_SCPRrRegenAvailTq_Nm"
  Bus Selector/13 -> [VINP_FrTMSpd_rpm]  "<VINP_FrTMSpd_rpm>"
  [VINP_CANMsgValidMCUNR1_flg] -> Switch4/2
  Bus Selector/41 -> [VINP_RrMCUTemp_C]  "<VINP_RrMCUTemp_C>"
  Switch7/1 -> [VTQD_SCPRrEDURealTMTq_Nm]  "VTQD_SCPRrEDURealTMTq_Nm"
  [VINP_RrRegenAvailTq_Nm] -> Switch5/3
  [VINP_RrTMSpd_rpm] -> Switch3/3
  [VINP_FrRegenAvailTq_Nm] -> Switch4/3
  [VINP_RrTMSpdNidec_rpm] -> Switch3/1
  [VINP_CANMsgValidMCUNR1_flg] -> Switch/2
  Switch2/1 -> [VTQD_SCPFrTMSpd_rpm]  "VTQD_SCPFrTMSpd_rpm"
  [VINP_FrTMSpd_rpm] -> Switch2/3
  [VINP_CANMsgValidMCUNR1_flg] -> Switch1/2
  Switch1/1 -> [VTQD_SCPRrEDURotateDirction_enum]  "VTQD_SCPRrEDURotateDirction_enum"
  [VINP_RrMotorAvailTq_Nm] -> Switch9/3
  Bus Selector/3 -> [VTQD_LowIdleAccPedal_flg]  "<VTQD_LowIdleAccPedal_flg>"
  Bus Selector/29 -> [VINP_MCUWarnF_enum]  "<VINP_MCUWarnF_enum>"
  Bus Selector/46 -> [VINP_SWC2RRegenDownSta_flg]  "<VINP_SWC2RRegenDownSta_flg>"
  Bus Selector/26 -> [VINP_RrMotorAvailTqNidec_Nm]  "<VINP_RrMotorAvailTqNidec_Nm>"
  Bus Selector/2 -> [VTQD_ActAPSPosn_pct]  "<VTQD_ActAPSPosn_pct>"
  [VINP_SWC2RRegenDownSta_flg] -> OR1/1
  Bus Selector/4 -> [VPMM_DrivetrainSelect_enum]  "<VPMM_DrivetrainSelect_enum>"
  Bus Selector/17 -> [VINP_FrRegenAvailTq_Nm]  "<VINP_FrRegenAvailTq_Nm>"
  Switch14/1 -> [VTQD_SCPFrMCUTemp_C]  "VTQD_SCPFrMCUTemp_C"
  [VINP_RrTMTempNidec_C] -> Switch17/1
  Bus Selector/24 -> [VINP_FrMotorAvailTqNidec_Nm]  "<VINP_FrMotorAvailTqNidec_Nm>"
  [VINP_CANMsgValidMCUNR1_flg] -> Switch5/2
  [VINP_MCUWarnRNidec_enum] -> Switch11/1
  Bus Selector/15 -> [VINP_RrTMSpd_rpm]  "<VINP_RrTMSpd_rpm>"
  Switch11/1 -> [VTQD_SCPMCUWarnR_enum]  "VTQD_SCPMCUWarnR_enum"
  Bus Selector/11 -> [VINP_RrEDURotateDirction_enum]  "<VINP_RrEDURotateDirction_enum>"
  [VINP_SWCRegenUp_flg] -> OR/1
  [VINP_FrTMSpdNidec_rpm] -> Switch2/1
  [VINP_CANMsgValidMCUNR1_flg] -> Switch2/2
  [VINP_FrMotorAvailTq_Nm] -> Switch8/3
  [VINP_CANMsgValidMCUNR1_flg] -> Switch3/2
  [VINP_RrRegenAvailTqNidec_Nm] -> Switch5/1
  [VINP_CANMsgValidMCUNR1_flg] -> Switch14/2
  Switch3/1 -> [VTQD_SCPRrTMSpd_rpm]  "VTQD_SCPRrTMSpd_rpm"
  [VINP_MCUWarnF_enum] -> Switch10/3
  [VINP_CANMsgValidMCUNR1_flg] -> Switch11/2
  [VINP_RrMCUDCBusVoltNidec_V] -> Switch13/1
  [VINP_SWCRegenDown_flg] -> OR1/2
  [VINP_CANMsgValidMCUNR1_flg] -> Switch15/2
  [VINP_FrEDURealTMTq_Nm] -> Switch6/3
  Switch4/1 -> [VTQD_SCPFrRegenAvailTq_Nm]  "VTQD_SCPFrRegenAvailTq_Nm"
  Bus Selector/5 -> [VINP_IVIPWModeReq_enum]  "<VINP_IVIPWModeReq_enum>"
  Switch16/1 -> [VTQD_SCPRrMCUTemp_C]  "VTQD_SCPRrMCUTemp_C"
  Bus Selector/20 -> [VINP_FrEDURealTMTqNidec_Nm]  "<VINP_FrEDURealTMTqNidec_Nm>"
  Bus Selector/19 -> [VINP_RrRegenAvailTq_Nm]  "<VINP_RrRegenAvailTq_Nm>"
  [VINP_CANMsgValidMCUNR1_flg] -> Switch10/2
  Bus Selector/12 -> [VINP_FrTMSpdNidec_rpm]  "<VINP_FrTMSpdNidec_rpm>"
  [VINP_CANMsgValidMCUNR1_flg] -> Switch6/2
  [VINP_FrEDURealTMTqNidec_Nm] -> Switch6/1
  Bus Selector/43 -> [VINP_RrTMTemp_C]  "<VINP_RrTMTemp_C>"
  Bus Selector/6 -> [VINP_IVISnowModeCmd_flg]  "<VINP_IVISnowModeCmd_flg>"
  Switch15/1 -> [VTQD_SCPFrTMTemp_C]  "VTQD_SCPFrTMTemp_C"
  BSCPIn_outputs/1 -> Bus Selector/1
  Equal20/1 -> [VTQD_RollRegenDisable_flg]  "VTQD_RollRegenDisable_flg"
  Constant2/1 -> Equal20/2
  [VTQD_RDCActive_enum] -> Equal20/1
  OR2/1 -> [VTQD_BrkSwSta_flg]  "VTQD_BrkSwSta_flg"
  LiuzgSwitch4/1 -> [VTQD_FrTMRotateDirction_enum]  "VTQD_FrTMRotateDirction_enum"
  GreaterThan/1 -> LiuzgSwitch2/2
  Constant20/1 -> GreaterThan3/2
  GreaterThan1/1 -> LiuzgSwitch3/2
  Constant11/1 -> LiuzgSwitch3/1
  Constant15/1 -> LiuzgSwitch9/3
  Constant18/1 -> GreaterThan1/2
  Constant19/1 -> LiuzgSwitch4/2
  Constant12/1 -> LiuzgSwitch3/3
  LiuzgSwitch8/1 -> LiuzgSwitch10/1
  LiuzgSwitch10/1 -> [VTQD_RrTMRotateDirction_enum]  "VTQD_RrTMRotateDirction_enum"
  Constant23/1 -> GreaterThan2/2
  GreaterThan3/1 -> LiuzgSwitch9/2
  GreaterThan2/1 -> LiuzgSwitch8/2
  LiuzgSwitch9/1 -> LiuzgSwitch8/3
  Constant14/1 -> LiuzgSwitch9/1
  LiuzgSwitch3/1 -> LiuzgSwitch2/3
  Constant28/1 -> LiuzgSwitch8/1
  Constant5/1 -> GreaterThan/2
  Constant22/1 -> LiuzgSwitch10/2
  Constant7/1 -> LiuzgSwitch2/1
  LiuzgSwitch2/1 -> LiuzgSwitch4/1
  [VINP_BrakeSWGPIO_flg] -> OR2/2
  [VTQD_SCPFrTMSpd_rpm] -> GreaterThan1/1, GreaterThan/1
  [VTQD_SCPRrTMSpd_rpm] -> GreaterThan3/1, GreaterThan2/1
  [VTQD_SCPFrEDURotateDirction_enum] -> LiuzgSwitch4/3
  Constant38/1 -> LiuzgSwitch13/3
  Equal7/1 -> Logical Operator5/1
  Equal9/1 -> Logical Operator5/2
  Constant37/1 -> Equal9/2
  Equal1/1 -> Logical Operator/2
  [VTQD_SCPFrTMSpd_rpm] -> Abs/1
  Logical Operator3/1 -> Logical Operator4/1
  Logical Operator5/1 -> Logical Operator4/2
  [VTQD_RrTMRotateDirction_enum] -> Equal9/1
  [VTQD_FrTMRotateDirction_enum] -> Equal3/1
  Equal/1 -> Logical Operator/1
  LiuzgSwitch11/1 -> [FrDirectionIndicator]  "FrDirectionIndicator"
  Gain2/1 -> [VTQD_RrShaftSpd_rpm]  "VTQD_RrShaftSpd_rpm"
  [RrDirectionIndicator] -> Product3/1
  [VTQD_SCPRrTMSpd_rpm] -> Abs1/1
  Constant34/1 -> LiuzgSwitch11/1
  Logical Operator4/1 -> LiuzgSwitch13/2
  Constant32/1 -> Equal3/2
  [FrDirectionIndicator] -> Product2/2
  Constant33/1 -> LiuzgSwitch11/3
  Constant10/1 -> Equal5/2
  Equal5/1 -> Logical Operator3/1
  Constant36/1 -> Equal7/2
  Equal6/1 -> Logical Operator3/2
  Product3/1 -> Gain2/1
  Product2/1 -> Gain/1
  Logical Operator2/1 -> Logical Operator1/2
  Constant31/1 -> Equal2/2
  Logical Operator1/1 -> LiuzgSwitch11/2
  Equal3/1 -> Logical Operator2/2
  Constant30/1 -> Equal1/2
  [VTQD_FrTMRotateDirction_enum] -> Equal1/1
  Equal2/1 -> Logical Operator2/1
  Constant29/1 -> Equal/2
  [VTQD_RrTMRotateDirction_enum] -> Equal6/1
  Gain/1 -> [VTQD_FrShaftSpd_rpm]  "VTQD_FrShaftSpd_rpm"
  Abs/1 -> Product2/1
  Constant39/1 -> LiuzgSwitch13/1
  Constant35/1 -> Equal6/2
  Logical Operator/1 -> Logical Operator1/1
  Abs1/1 -> Product3/2
  LiuzgSwitch13/1 -> [RrDirectionIndicator]  "RrDirectionIndicator"
  [VTQD_GearActualPosn_enum] -> Equal/1
  [VPMM_DrivetrainSelect_enum] -> Equal4/1
  [VPMM_DrivetrainSelect_enum] -> Equal8/1
  Equal8/1 -> LiuzgSwitch7/2
  Constant21/1 -> Equal8/2
  [VTQD_FrShaftSpd_rpm] -> LiuzgSwitch7/1
  Constant6/1 -> Equal4/2
  [VTQD_FrTMRotateDirction_enum] -> LiuzgSwitch12/1
  [VTQD_RrTMRotateDirction_enum] -> LiuzgSwitch12/3
  Equal4/1 -> LiuzgSwitch12/2
  [VTQD_RrShaftSpd_rpm] -> LiuzgSwitch7/3
  LiuzgSwitch7/1 -> [VTQD_TqTargetShaftSpd_rpm]  "VTQD_TqTargetShaftSpd_rpm"
  LiuzgSwitch12/1 -> [VTQD_TMRotateDirction_enum]  "VTQD_TMRotateDirction_enum"
  Constant47/1 -> Equal21/2
  Constant69/1 -> LiuzgSwitch22/1
  Equal21/1 -> LiuzgSwitch21/2
  Constant71/1 -> LiuzgSwitch21/1
  LiuzgSwitch22/1 -> LiuzgSwitch21/3
  [VINP_IVIPWModeReq_enum] -> Equal22/1
  [VINP_IVISnowModeCmd_flg] -> LiuzgSwitch1/2
  Constant17/1 -> Switch22/1
  Constant16/1 -> Switch22/2
  [VTQD_LimpHomeAct_flg] -> LiuzgSwitch24/2  "VTQD_LimpHomeAct_flg"
  Constant130/1 -> LiuzgSwitch1/1
  LiuzgSwitch1/1 -> LiuzgSwitch24/3
  Constant132/1 -> LiuzgSwitch24/1
  [VINP_IVIPWModeReq_enum] -> Equal21/1
  Equal22/1 -> LiuzgSwitch22/2
  LiuzgSwitch24/1 -> Switch22/3
  Constant70/1 -> Equal22/2
  LiuzgSwitch21/1 -> LiuzgSwitch1/3
  Constant46/1 -> LiuzgSwitch22/3
  Switch22/1 -> [VTQD_EVDriveMode_enum]  "VTQD_EVDriveMode_enum"
  Constant75/1 -> Equal14/2
  Constant76/1 -> Equal15/2
  [VPMM_DrivetrainSelect_enum] -> Equal15/1
  FWDMCUReadyExt_flg/1(VTQD_FWDMCUReadyExt_flg) -> Merge/2
  [VPMM_DrivetrainSelect_enum] -> Equal14/1
  [VTQD_SCPMCUWarnR_enum] -> RWDMCUReadyExt_flg/1(VINP_RrMCUErr_enum)
  [VTQD_SCPMCUWarnF_enum] -> FWDMCUReadyExt_flg/1(VINP_FrMCUErr_enum)
  Equal15/1 -> If/2
  Equal14/1 -> If/1
  RWDMCUReadyExt_flg/1(VTQD_RWDMCUReadyExt_flg) -> Merge/3
  If/2 -> FWDMCUReadyExt_flg/Action
  [VPMM_DrivetrainSelect_enum] -> Equal16/1
  If/3 -> RWDMCUReadyExt_flg/Action
  Constant72/1 -> Equal16/2
  Merge/1 -> [VTQD_MCUReady4Ext_flg]  "VTQD_MCUReady4Ext_flg"
  [VTQD_SCPMCUWarnR_enum] -> AWDMCUReadyExt_flg/2(VINP_RrMCUErr_enum)
  If/1 -> AWDMCUReadyExt_flg/Action
  [VTQD_SCPMCUWarnF_enum] -> AWDMCUReadyExt_flg/1(VINP_FrMCUErr_enum)
  Equal16/1 -> If/3
  AWDMCUReadyExt_flg/1(VTQD_AWDMCUReadyExt_flg) -> Merge/1
  [VTQD_LowIdleAccPedal_flg] -> Switch31/3
  AND3/1 -> Switch32/2
  [VTQD_RegenModeChange_flg] -> AND3/2
  [VTQD_RgnChgReset_flg] -> Delay3/1
  [VTQD_ActAPSPosn_pct] -> Add/1
  Constant73/1 -> Relational Operator1/2
  Delay3/1 -> SR_Latch/2
  Abs2/1 -> Relational Operator1/1
  Delay2/1 -> Switch29/1
  Constant1/1 -> Switch31/2
  Switch32/1 -> Delay1/1, [VTQD_RegenMode_enum]  "VTQD_RegenMode_enum"
  Switch29/1 -> [VTQD_RgnModeChgAPSPosn_pct], Delay2/1  "VTQD_RgnModeChgAPSPosn_pct"
  Delay1/1 -> Switch32/1
  Detect Change/1 -> SR_Latch/1
  Switch31/1 -> [VTQD_RgnChgReset_flg]  "VTQD_RgnChgReset_flg"
  Constant74/1 -> AND3/1
  [VTQD_RgnModeChgAPSPosn_pct] -> Add/2
  Add/1 -> Abs2/1
  [VTQD_RegenModeChange_flg] -> Switch29/2
  [VTQD_FDCVCURegenMode_enum] -> Detect Change/1
  Relational Operator1/1 -> Switch31/1
  [VTQD_ActAPSPosn_pct] -> Switch29/3
  SR_Latch/1 -> [VTQD_RegenModeChange_flg]  "VTQD_RegenModeChange_flg"
  [VTQD_FDCVCURegenMode_enum] -> Switch32/3
  [VTQD_SCPRrEDURotateDirction_enum] -> LiuzgSwitch10/3
  [VTQD_RollRegenDisable_flg] -> Bus Creator/2
  [VTQD_ShiftGearPosn_enum] -> Bus Creator/4
  [VTQD_TqTargetShaftSpd_rpm] -> Bus Creator/5
  [VTQD_TMRotateDirction_enum] -> Bus Creator/6
  [VTQD_EVDriveMode_enum] -> Bus Creator/7
  [VTQD_MCUReady4Ext_flg] -> Bus Creator/8
  [VTQD_RegenMode_enum] -> Bus Creator/9
  Bus Creator/1 -> BSignalConvert_outputs/1
  [VTQD_BrkSwSta_flg] -> Bus Creator/3
  [VTQD_FrShaftSpd_rpm] -> Bus Creator/10
  [VTQD_RrShaftSpd_rpm] -> Bus Creator/11
  [VTQD_LowIdleAccPedal_flg] -> Bus Creator/1
  [VTQD_LimpHomeAct_flg] -> Bus Creator/12  "VTQD_LimpHomeAct_flg"
  [VTQD_RDCActive_enum] -> Bus Creator/13
  [VTQD_SCPFrRegenAvailTq_Nm] -> Bus Creator/14
  [VTQD_SCPRrRegenAvailTq_Nm] -> Bus Creator/15
  [VTQD_SCPFrMotorAvailTq_Nm] -> Bus Creator/16
  [VTQD_SCPRrMotorAvailTq_Nm] -> Bus Creator/17
  [VTQD_SCPFrMCUDCBusVolt_V] -> Bus Creator/18
  [VTQD_SCPRrMCUDCBusVolt_V] -> Bus Creator/19
  [VTQD_SCPFrMCUTemp_C] -> Bus Creator/20
  [VTQD_SCPFrTMTemp_C] -> Bus Creator/21
  [VTQD_SCPRrMCUTemp_C] -> Bus Creator/22
  [VTQD_SCPRrTMTemp_C] -> Bus Creator/23
  [VTQD_SCPSWCRegenUp_flg] -> Bus Creator/24
  [VTQD_SCPSWCRegenDown_flg] -> Bus Creator/25
  Bus Selector/51 -> [VINP_BrkSwStaSW_flg]  "<VINP_BrkSwSta_flg>"
  [VINP_BrkSwStaSW_flg] -> OR2/1
  BFunction_outputs/1 -> Bus Selector1/1
  Bus Selector1/1 -> [VTQD_GearActualPosn_enum]  "<VTQD_GearActualPosn_enum>"
  Bus Selector1/2 -> [VTQD_FDCVCURegenMode_enum]  "<VTQD_FDCVCURegenMode_enum>"
  [VTQD_SCPFrEDURotateDirction_enum] -> Bus Creator/26
  [VTQD_SCPRrEDURotateDirction_enum] -> Bus Creator/27
  [VTQD_SCPFrTMSpd_rpm] -> Bus Creator/28
  [VTQD_SCPRrTMSpd_rpm] -> Bus Creator/29
  [VTQD_SCPFrEDURealTMTq_Nm] -> Bus Creator/30
  [VTQD_SCPRrEDURealTMTq_Nm] -> Bus Creator/31
  [VTQD_SCPMCUWarnF_enum] -> Bus Creator/32
  [VTQD_SCPMCUWarnR_enum] -> Bus Creator/33
  Switch28/1 -> [VTQD_IVIPwrLockSta_enum]  "VTQD_IVIPwrLockSta_enum"
  Constant81/1 -> Equal31/2
  OR4/1 -> AND4/1
  [VTQD_IVIPwrLock_flg] -> Switch28/2
  [VTQD_GearActualPosn_enum] -> Equal31/1
  Delay4/1 -> AND4/2
  Constant97/1 -> Switch28/1
  AND4/1 -> [VTQD_IVIPwrLock_flg]  "VTQD_IVIPwrLock_flg"
  Equal31/1 -> Delay4/1
  Constant98/1 -> Switch28/3
  [VTQD_IVIPwrLock_flg] -> Bus Creator/34
  [VTQD_IVIPwrLockSta_enum] -> Bus Creator/35
  [VTQD_TMRotateDirction_enum] -> Equal18/1
  Constant9/1 -> Equal17/2
  Equal17/1 -> Logical Operator6/1
  Constant27/1 -> LiuzgSwitch5/3
  Constant13/1 -> Equal18/2
  Logical Operator8/1 -> Logical Operator7/2
  Constant24/1 -> Equal19/2
  Logical Operator6/1 -> Logical Operator7/1
  Constant25/1 -> Equal23/2
  Equal23/1 -> Logical Operator8/2
  Logical Operator7/1 -> LiuzgSwitch5/2
  [VTQD_GearActualPosn_enum] -> Delay5/1
  LiuzgSwitch5/1 -> [VTQD_VehActSpdGain_gain]  "VTQD_VehActSpdGain_gain"
  Equal18/1 -> Logical Operator6/2
  [VTQD_GearActualPosn_enum] -> Delay6/1
  Constant26/1 -> LiuzgSwitch5/1
  [VTQD_TMRotateDirction_enum] -> Equal23/1
  Equal19/1 -> Logical Operator8/1
  Bus Selector/1 -> [task_time_s]  "<task_time_s>"
  Bus Selector/52 -> [VVMC_APSActive_flg]  "<VVMC_APSActive_flg>"
  Bus Selector/53 -> [VINP_VehSpeed_kph]  "<VINP_VehSpeed_kph>"
  [VTQD_VehActSpd_kph] -> Bus Creator/36
  Delay5/1 -> Equal17/1
  Delay6/1 -> Equal19/1
  Equal25/1 -> OR3/1
  [VTQD_GearActualPosn_enum] -> Equal25/2, Equal24/1
  Constant42/1 -> Equal24/2
  Constant43/1 -> Equal25/1
  Equal24/1 -> OR3/2
  NOT1/1 -> [VTQD_NoSuitbleGear_flg]  "VTQD_NoSuitbleGear_flg"
  OR3/1 -> NOT1/1
  [VTQD_NoSuitbleGear_flg] -> Bus Creator/37
  [VINP_IVISnowModeCmd_flg] -> Switch27/2
  Ground1/1 -> [VINP_SCPSystemMode_enum]
  Equal26/1 -> Switch25/2
  Constant49/1 -> Equal27/2
  Constant44/1 -> Equal28/2
  [VTQR_EVDriveMode_enum] -> Equal27/1
  Constant59/1 -> Relational Operator4/2
  [VINP_VehSpeed_kph] -> Relational Operator6/1
  [VTQD_GearActualPosn_enum] -> Equal26/1
  RegenLV_inc1/1 -> Equal29/2
  [VDHP_ActAPSPosn_pct] -> Relational Operator4/1
  Relational Operator4/1 -> AND/1
  RegenLV_inc6/1 -> Switch25/1
  Constant45/1 -> Switch26/1
  Relational Operator6/1 -> AND/2
  Switch26/1 -> [VTQR_RampTqCMDGain_c]  "VTQR_RampTqCMDGain_c"
  Constant61/1 -> Switch26/3
  [VTQD_RegenMode_enum] -> Equal28/1
  Switch27/1 -> Switch25/3
  RegenLV_inc2/1 -> Switch27/1
  RegenLV_inc5/1 -> Equal26/2
  [VINP_SCPSystemMode_enum] -> Terminator2/1
  Equal29/1 -> Switch26/2
  Equal27/1 -> AND/3
  Constant60/1 -> Relational Operator6/2
  [VTQD_GearActualPosn_enum] -> Equal29/1
  AND/1 -> [VTQR_LaunchEn_flg]  "VTQR_LaunchEn_flg"
  [VTQD_EVDriveMode_enum] -> Switch27/3
  Equal28/1 -> AND/4
  Switch25/1 -> [VTQR_EVDriveMode_enum]  "VTQR_EVDriveMode_enum"
  Bus Selector/54 -> [VDHP_ActAPSPosn_pct]  "<VTQD_ActAPSPosn_pct>"
  [VTQR_LaunchEn_flg] -> Bus Creator/38
  [VTQR_RampTqCMDGain_c] -> Bus Creator/39
  [VTQR_EVDriveMode_enum] -> Bus Creator/40
  [VTQD_OPDHoldForceEn_flg] -> OR6/1
  Constant52/1 -> Equal48/2
  [VINP_EPBSta_enum] -> Equal48/1
  OR6/1 -> AND1/2
  Equal13/1 -> AND1/1
  [VTQD_ShiftGearPosn_enum] -> Delay7/1
  Equal48/1 -> OR6/2
  Delay7/1 -> Switch18/3
  Constant58/1 -> Equal13/2
  Constant51/1 -> Switch18/1
  Constant54/1 -> Equal11/2
  Constant56/1 -> Equal12/2
  Switch18/1 -> Switch19/3
  [VTQD_GearActualPosn_enum] -> Equal11/1
  [VTQD_GearActualPosn_enum] -> Equal10/1
  Switch20/1 -> Switch21/3
  [VTQD_GearActualPosn_enum] -> Equal13/1
  Constant57/1 -> Switch21/1
  [VTQD_GearActualPosn_enum] -> Equal12/1
  Equal12/1 -> Switch20/2
  Equal11/1 -> Switch19/2
  Switch21/1 -> [VTQD_ShiftGearPosn_enum]  "VTQD_ShiftGearPosn_enum"
  Constant55/1 -> Switch20/1
  Constant53/1 -> Equal10/2
  Switch19/1 -> Switch20/3
  Constant50/1 -> Switch19/1
  AND1/1 -> Switch21/2
  Equal10/1 -> Switch18/2
  Constant116/1 -> Data Type Conversion8/1
  Data Type Conversion3/1 -> Equal34/2
  Data Type Conversion8/1 -> Equal47/2
  [VINP_DIDGetExhibitMode_enum] -> Equal34/1
  Equal34/1 -> OR4/1
  Constant96/1 -> Data Type Conversion3/1
  Equal47/1 -> OR4/2
  [VINP_DIDGetExhibitMode_enum] -> Equal47/1
  Bus Selector/55 -> [VINP_DIDGetExhibitMode_enum]  "<VINP_DIDGetExhibitMode_enum>"
  [VTQD_RPM2VehSpd_kph] -> Switch23/1
  Constant48/1 -> AND10/1
  [VTQD_VehActSpdGain_gain] -> Product/1
  [VINP_VehSpeed_kph] -> Product/2
  Relay1/1 -> AND9/2
  Switch23/1 -> [VTQD_VehActSpd_kph]  "VTQD_VehActSpd_kph"
  AND10/1 -> AND9/1
  Product/1 -> Switch23/3
  AND9/1 -> Switch23/2
  [VVMC_APSActive_flg] -> AND10/2
  [VINP_VehSpeed_kph] -> Relay1/1
  [VTQD_ActSpdCalInp_rpm] -> Product1/1
  Constant4/1 -> Product1/3
  Product1/1 -> FirstOrderFilter/1
  Constant3/1 -> Product1/2
  Constant40/1 -> FirstOrderFilter/3
  Constant8/1 -> Product1/4
  FirstOrderFilter/1 -> [VTQD_RPM2VehSpd_kph]  "VTQD_RPM2VehSpd_kph"
  [task_time_s] -> FirstOrderFilter/2
  Switch30/1 -> [VTQD_ActSpdCalInp_rpm]  "VTQD_ActSpdCalInp_rpm"
  [VTQR_NoABSFEDUWhlTqReq_Nm] -> Delay/1
  Relational Operator2/1 -> Switch24/2
  Constant66/1 -> Equal51/2
  [VPMM_DrivetrainSelect_enum] -> Equal51/1
  Constant41/1 -> AND18/2
  [VTQD_TqTargetShaftSpd_rpm] -> Switch30/3
  AND18/1 -> Switch30/2
  Abs4/1 -> Relational Operator2/2
  Abs3/1 -> Relational Operator2/1
  [VTQR_NoABSREDUWhlTqReq_Nm] -> Delay8/1
  Equal51/1 -> AND18/1
  Switch24/1 -> Switch30/1
  Bus Selector/56 -> [VINP_EPBSta_enum]  "<VINP_EPBSta_enum>"
  [VTQD_GearActualPosn_enum] -> Equal2/1
  [VTQD_GearActualPosn_enum] -> Equal5/1
  [VTQD_GearActualPosn_enum] -> Equal7/1
  BMain_outputs/1 -> Bus Selector2/1
  [VTQD_RrShaftSpd_rpm] -> Switch24/3
  [VTQD_FrShaftSpd_rpm] -> Switch24/1
  Bus Selector2/1 -> [VTQR_NoABSFEDUWhlTqReq_Nm]  "<VTQR_NoABSFEDUWhlTqReq_Nm>"
  Bus Selector2/2 -> [VTQR_NoABSREDUWhlTqReq_Nm]  "<VTQR_NoABSREDUWhlTqReq_Nm>"
  Delay/1 -> Abs3/1
  Delay8/1 -> Abs4/1
  Bus Selector1/3 -> [VTQD_OPDHoldForceEn_flg]  "<VTQD_OPDHoldForceEn_flg>"
  [VINP_IVICreepSWReq_flg] -> Switch33/3
  Switch33/1 -> [VTQD_CreepON_flg]  "VTQD_CreepON_flg"
  Constant/1 -> Switch33/2
  Constant62/1 -> Switch33/1
  [VTQD_CreepON_flg] -> Bus Creator/41
  Bus Selector/57 -> [VINP_IVICreepSWReq_flg]  "<VINP_IVICreepSWReq_flg>"
